simulink model "example2_old"  (Simulink 7.1)
settings: Solver=ode4  StartTime=0.0  StopTime=20  FixedStep=0.01  RelTol=1e-3
InitFcn:
  | Ku = 3.665;
  | Tu = 2.06;
  | Kpmin = 0.32*Ku;
  | Kpmax = 0.6*Ku;
  | Kdmin = 0.08*Ku*Tu;
  | Kdmax = 0.15*Ku*Tu;
  | fuzzy_pid = readfis('fuzzy_pid');
libraries: fuzblock x1
settings Model: Creator=sahandar  LastModifiedBy=smk
settings OptimizationCC: ExpressionDepthLimit=128  InitFltsAndDblsToZero=off
settings DebuggingCC: SolverPrmCheckMsg=none  FcnCallInpInsideContextMsg=Enable All  StateNameClashWarn=none  StrictBusMsg=ErrorLevel1
settings CodeAppCC: CustomSymbolStrType=$N$R$M_T
settings GRTTargetCC: TargetFunctionLibrary=C89/C90 (ANSI)  CPPClassGenCompliant=off

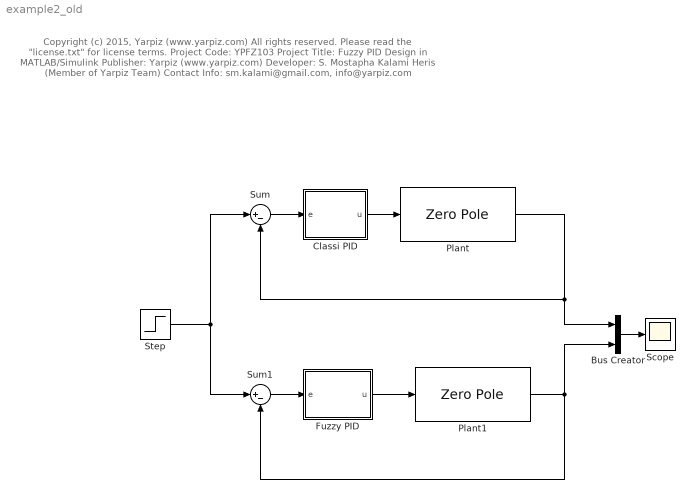
== system example2_old ==
  note: Copyright (c) 2015, Yarpiz (www.yarpiz.com)
      | All rights reserved. Please read the "license.txt" for license terms.
      | Project Code: YPFZ103
      | Project Title: Fuzzy PID Design in MATLAB/Simulink
      | Publisher: Yarpiz (www.yarpiz.com)
      | Developer: S. Mostapha Kalami Heris (Member of Yarpiz Team)
      | Contact Info: sm.kalami@gmail.com, info@yarpiz.com
  Bus Creator : BusCreator  Inputs=2
  Classi PID : Subsystem
  Fuzzy PID : Subsystem
  Plant : ZeroPole  Zeros=[]  Poles=[-0.5 -0.8200 + 2.7899i -0.8200 - 2.7899i]  Gain=4.228
  Plant1 : ZeroPole  Zeros=[]  Poles=[-0.5 -0.8200 + 2.7899i -0.8200 - 2.7899i]  Gain=4.228
  Scope : Scope
      settings: YMin=0.00525  YMax=0.009
  Step : Step  Time=0  SampleTime=0
  Sum : Sum  Inputs=|+-
  Sum1 : Sum  Inputs=|+-
  wires:
  Classi PID/1(u) -> Plant/1
  Sum/1 -> Classi PID/1(e)
  Step/1 -> Sum/1, Sum1/1
  Plant/1 -> Sum/2, Bus Creator/1
  Plant1/1 -> Sum1/2, Bus Creator/2
  Bus Creator/1 -> Scope/1
  Sum1/1 -> Fuzzy PID/1(e)
  Fuzzy PID/1(u) -> Plant1/1

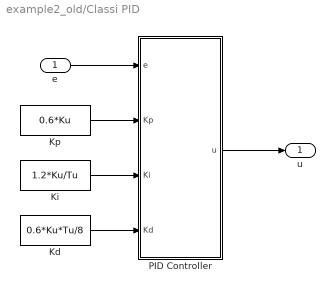
== system example2_old/Classi PID ==
  e : Inport
  Kd : Constant  Value=0.6*Ku*Tu/8
  Ki : Constant  Value=1.2*Ku/Tu
  Kp : Constant  Value=0.6*Ku
  PID Controller : Subsystem
  u : Outport
  wires:
  Kd/1 -> PID Controller/4(Kd)
  PID Controller/1(u) -> u/1
  e/1 -> PID Controller/1(e)
  Kp/1 -> PID Controller/2(Kp)
  Ki/1 -> PID Controller/3(Ki)

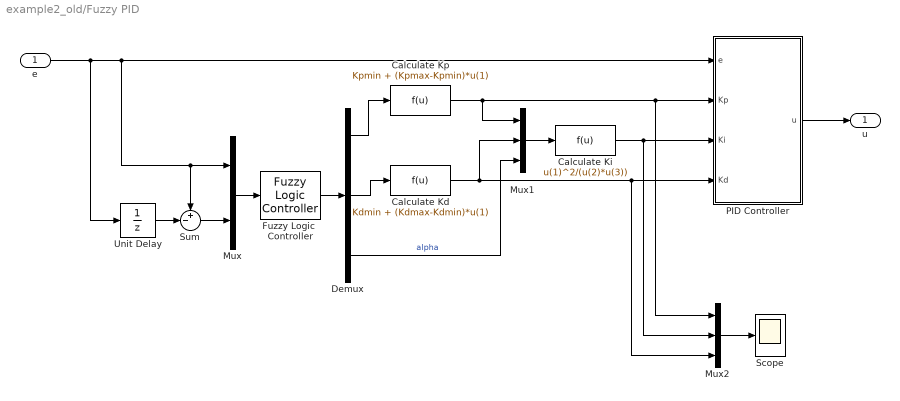
== system example2_old/Fuzzy PID ==
  e : Inport
  Calculate Kd : Fcn  Expr=Kdmin + (Kdmax-Kdmin)*u(1)
  Calculate Ki : Fcn  Expr=u(1)^2/(u(2)*u(3))
  Calculate Kp : Fcn  Expr=Kpmin + (Kpmax-Kpmin)*u(1)
  Demux : Demux  Outputs=3
  Fuzzy Logic  Controller : fuzblock/Fuzzy Logic  Controller  fis=fuzzy_pid
  Mux : Mux  Inputs=2
  Mux1 : Mux  Inputs=3
  Mux2 : Mux  Inputs=3
  PID Controller : Subsystem
  Scope : Scope
  Sum : Sum  Inputs=+-|
  Unit Delay : UnitDelay  SampleTime=-1
  u : Outport
  wires:
  e/1 -> Unit Delay/1, PID Controller/1(e), Sum/1, Mux/1
  Mux/1 -> Fuzzy Logic  Controller/1
  Fuzzy Logic  Controller/1 -> Demux/1
  Demux/1 -> Calculate Kp/1
  Calculate Kp/1 -> PID Controller/2(Kp), Mux2/1, Mux1/1
  Demux/2 -> Calculate Kd/1
  Calculate Kd/1 -> Mux1/2, PID Controller/4(Kd), Mux2/3
  Calculate Ki/1 -> PID Controller/3(Ki), Mux2/2
  Mux1/1 -> Calculate Ki/1
  Sum/1 -> Mux/2
  Unit Delay/1 -> Sum/2
  Mux2/1 -> Scope/1
  PID Controller/1(u) -> u/1
  Demux/3 -> Mux1/3  "alpha"

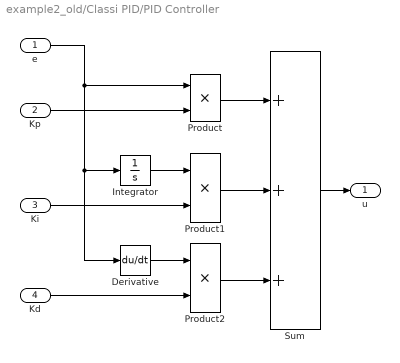
== system example2_old/Classi PID/PID Controller ==
  e : Inport
  Kp : Inport  Port=2
  Ki : Inport  Port=3
  Kd : Inport  Port=4
  Derivative : Derivative
  Integrator : Integrator
  Product : Product
  Product1 : Product
  Product2 : Product
  Sum : Sum  Inputs=3
  u : Outport
  wires:
  Sum/1 -> u/1
  Product/1 -> Sum/1
  Kp/1 -> Product/2
  e/1 -> Derivative/1, Integrator/1, Product/1
  Ki/1 -> Product1/2
  Integrator/1 -> Product1/1
  Product1/1 -> Sum/2
  Product2/1 -> Sum/3
  Kd/1 -> Product2/2
  Derivative/1 -> Product2/1

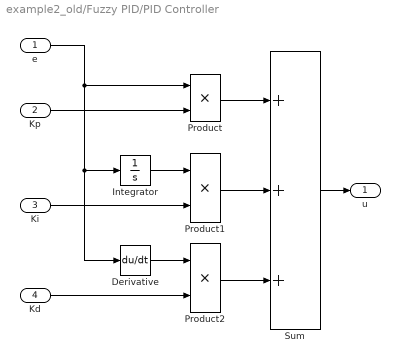
== system example2_old/Fuzzy PID/PID Controller ==
  e : Inport
  Kp : Inport  Port=2
  Ki : Inport  Port=3
  Kd : Inport  Port=4
  Derivative : Derivative
  Integrator : Integrator
  Product : Product
  Product1 : Product
  Product2 : Product
  Sum : Sum  Inputs=3
  u : Outport
  wires:
  Sum/1 -> u/1
  Product/1 -> Sum/1
  Kp/1 -> Product/2
  e/1 -> Derivative/1, Integrator/1, Product/1
  Ki/1 -> Product1/2
  Integrator/1 -> Product1/1
  Product1/1 -> Sum/2
  Product2/1 -> Sum/3
  Kd/1 -> Product2/2
  Derivative/1 -> Product2/1
